simulink model "PLL_linecut"  (R2025a)
settings: Solver=FixedStepAuto  StartTime=0.0  StopTime=t_sim_start+t_end  FixedStep=Ts  RelTol=1e-3
values from neighbouring files (symbols this model uses):
  C_dc = 2.25    [PLLpara.m]
  Cf1 = 0.01    [PLLpara.m]
  Cf2 = 0.01    [PLLpara.m]
  dt_sag = t_c    [GFMPara.m]    (also in GFMPara_exp.m; PLLpara.m; VFMPara.m; VFMPara_exp.m)
  f_switching = 20e3    (= 20000)    [GFMPara_exp.m]    (also in PLLpara.m = 10000; VFMPara_exp.m)
  Id0 = Id    [PLLpara.m]
  Iq01 = 0    [PLLpara.m]
  Iq02 = (Ug*cos(asin((Xg*Id+Rg*Iq)/Ug))+Id*Rg-Iq*Xg)*Cf2+Iq    [PLLpara.m]
  ki_pll1 = ki    [PLLpara.m]
  kp_pll1 = kp    [PLLpara.m]
  Lc = 1e-9    (= 1e-09)    [GFMPara.m]    (also in GFMPara_exp.m; PLLpara.m; VFMPara.m; VFMPara_exp.m)
  Lf = 0.0592    [GFMPara.m]    (also in GFMPara_exp.m; PLLpara.m = 0.05; VFMPara.m = 0.05; VFMPara_exp.m = 0.05)
  Lg1 = X1    [PLLpara.m]    (also in VFMPara.m; VFMPara_exp.m)
  Lgg = Xgg    [PLLpara.m]    (also in VFMPara.m; VFMPara_exp.m)
  Rf = 1e-3    (= 0.001)    [PLLpara.m]
  Rg1 = R1    [PLLpara.m]    (also in VFMPara.m; VFMPara_exp.m = 4*R1/5)
  Rgg = Rgg    [PLLpara.m]    (also in VFMPara.m; VFMPara_exp.m)
  Sbase = 1    [GFMPara.m]    (also in GFMPara_exp.m; PLLpara.m; VFMPara.m; VFMPara_exp.m)
  t0 = t_sim_start +t_start    [PLLpara.m]    (also in VFMPara_exp.m)
  t0_sag = t_sim_start +t_start    [GFMPara.m]    (also in GFMPara_exp.m; PLLpara.m = 20; VFMPara.m; VFMPara_exp.m = 20)
  Tc = 1/f_switching    (= 5e-05)    [GFMPara_exp.m]    (also in PLLpara.m = 0.0001; VFMPara_exp.m)
  tc = t_c    [PLLpara.m]    (also in VFMPara_exp.m)
  Ts = 1/Fs    (= 1e-05)    [GFMPara.m]    (also in GFMPara_exp.m = 1e-06; PLLpara.m = 1e-06; VFMPara.m = 5e-06; VFMPara_exp.m = 1e-06)
  v_sag = Ug_fault    [GFMPara.m]    (also in GFMPara_exp.m; PLLpara.m; VFMPara.m; VFMPara_exp.m)
  Vbase = 1    [GFMPara.m]    (also in GFMPara_exp.m; PLLpara.m; VFMPara.m; VFMPara_exp.m)
  Vdc = 2.5    [PLLpara.m]
  w_i_GFL1 = 1100 *2*pi    (= 6911.5038379)    [PLLpara.m]
  w_i_GFL2 = 1100 *2*pi    (= 6911.5038379)    [PLLpara.m]
  w_pll1 = 10 *2*pi    (= 62.8318530718)    [PLLpara.m]
  w_tau1 = 1500 *2*pi    (= 9424.77796077)    [PLLpara.m]
  Wbase = 2*pi*50    (= 314.159265359)    [GFMPara.m]    (also in GFMPara_exp.m; PLLpara.m; VFMPara.m; VFMPara_exp.m)
  Zbase = Vbase/Ibase    (= 1)    [GFMPara.m]    (also in GFMPara_exp.m; PLLpara.m; VFMPara.m; VFMPara_exp.m)
undefined symbols (not defined in the file or in its folder): DiscIntNeverNeededParam, dspblkCoreblockFVToolHelper, gcbh, initial, position, postfault_SEP, sigbuilder_block, w_max, w_min, Ws
libraries: spsVoltageMeasurementLib x80, spsCurrentMeasurementLib x75, spsIdealSwitchLib x30, spsThreePhaseSeriesRLCBranchLib x21, spsControlledVoltageSourceLib x18, spsSeriesRLCBranchLib x14, powerlib_extras x10, spsHalfBridgeConverterLib x6, spsThreePhaseBreakerLib x6, spsDCVoltageSourceLib x4, simulink x3, spsThreePhaseFaultLib x3
(part 5 of 6)

== system PLL_linecut/Grid-Following Inverter (Simulink Block)3/inverter2 ==
  G : Inport
  block : Inport  Port=2
  Demux : Demux  Outputs=3
  NPC : Subsystem
  NPC1 : Subsystem
  NPC2 : Subsystem
  DC+ : PMIOPort  Tag=PMCPort  Side=Left
  N : PMIOPort  Tag=PMCPort  Port=2  Side=Left
  DC- : PMIOPort  Tag=PMCPort  Port=3  Side=Left
  A : PMIOPort  Tag=PMCPort  Port=4  Side=Right
  B : PMIOPort  Tag=PMCPort  Port=5  Side=Right
  C : PMIOPort  Tag=PMCPort  Port=6  Side=Right
  wires:
  G/1 -> Demux/1
  Demux/1 -> NPC/1(gate)
  Demux/2 -> NPC1/1(gate)
  Demux/3 -> NPC2/1(gate)
  block/1 -> NPC/2(block), NPC2/2(block), NPC1/2(block)
  connections:
  C/RConn1 -- NPC2/RConn1
  NPC1/RConn1 -- B/RConn1
  A/RConn1 -- NPC/RConn1
  DC+/RConn1 -- NPC2/LConn1 -- NPC1/LConn1 -- NPC/LConn1
  NPC/LConn3 -- NPC1/LConn3 -- NPC2/LConn3 -- DC-/RConn1
  NPC/LConn2 -- NPC2/LConn2 -- NPC1/LConn2 -- N/RConn1

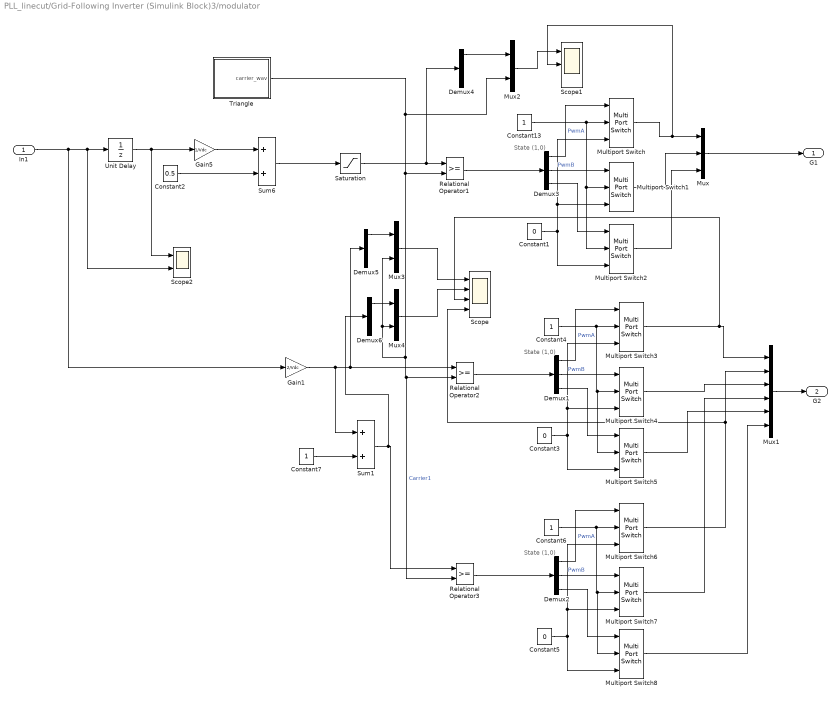
== system PLL_linecut/Grid-Following Inverter (Simulink Block)3/modulator ==
  note: State
      | (1,0)
  note: State
      | (1,0)
  note: State
      | (1,0)
  In1 : Inport  SampleTime=Ts
  Constant1 : Constant  Value=0
  Constant{4,6..7,13} (4 alike) : Constant
  Constant2 : Constant  Value=0.5
  Constant3 : Constant  Value=0
  Constant5 : Constant  Value=0
  Demux{1..6} (6 alike) : Demux  Outputs=3
      settings: DisplayOption=none
  Gain1 : Gain  Gain=2/Vdc
  Gain5 : Gain  Gain=1/Vdc
  Multiport Switch{,1..8} (9 alike) : MultiPortSwitch  DataPortOrder=Specify indices  DataPortIndices={1,0}  SaturateOnIntegerOverflow=off
  Mux : Mux  Inputs=[1 1 1]
  Mux1 : Mux  Inputs=6
  Mux2 : Mux  Inputs=2
  Mux3 : Mux  Inputs=2
  Mux4 : Mux  Inputs=2
  Relational Operator1 : RelationalOperator  OutDataTypeStr=float('double')
  Relational Operator2 : RelationalOperator  OutDataTypeStr=float('double')
  Relational Operator3 : RelationalOperator  OutDataTypeStr=float('double')
  Saturation : Saturate  UpperLimit=1  LowerLimit=0
  Scope : Scope  NumInputPorts=4
      settings: ActiveDisplayYMinimum=-0.88942  ActiveDisplayYMaximum=1.38183
  Scope1 : Scope  NumInputPorts=3
      settings: ActiveDisplayYMinimum=-0.044652738883298015  ActiveDisplayYMaximum=0.93484284042216537  DataLoggingVariableName=ScopeData6
  Scope2 : Scope  NumInputPorts=2
      settings: ActiveDisplayYMinimum=-0.80845  ActiveDisplayYMaximum=0.88075
  Sum1 : Sum  InputSameDT=on  SaturateOnIntegerOverflow=on  OutDataTypeStr=Inherit: Same as first input
  Sum6 : Sum  InputSameDT=on  SaturateOnIntegerOverflow=on  OutDataTypeStr=Inherit: Same as first input
  Triangle : Subsystem
  Unit Delay : UnitDelay  SampleTime=Tc  HasFrameUpgradeWarning=on
  G1 : Outport
  G2 : Outport  Port=2
  wires:
  Triangle/1(carrier_wav) -> Mux2/2, Mux4/2, Mux3/2, Relational Operator3/2, Relational Operator2/2, Relational Operator1/2  "Carrier1"
  Relational Operator1/1 -> Demux3/1
  Multiport Switch/1 -> Scope1/2, Mux/1
  Multiport Switch2/1 -> Mux/3
  Multiport Switch1/1 -> Mux/2
  Demux3/1 -> Multiport Switch/1  "PwmA"
  Demux3/2 -> Multiport Switch1/1  "PwmB"
  Demux3/3 -> Multiport Switch2/1
  Constant13/1 -> Multiport Switch2/2, Multiport Switch1/2, Multiport Switch/2
  Constant1/1 -> Multiport Switch1/3, Multiport Switch/3, Multiport Switch2/3
  Mux/1 -> G1/1
  Gain5/1 -> Sum6/1
  Constant2/1 -> Sum6/2
  In1/1 -> Scope2/2, Unit Delay/1, Gain1/1
  Demux1/3 -> Multiport Switch5/1
  Demux1/2 -> Multiport Switch4/1  "PwmB"
  Constant4/1 -> Multiport Switch5/2, Multiport Switch4/2, Multiport Switch3/2
  Multiport Switch5/1 -> Mux1/5
  Demux1/1 -> Multiport Switch3/1  "PwmA"
  Multiport Switch4/1 -> Mux1/3
  Constant3/1 -> Multiport Switch4/3, Multiport Switch3/3, Multiport Switch5/3
  Multiport Switch3/1 -> Scope/3, Mux1/1
  Relational Operator2/1 -> Demux1/1
  Constant5/1 -> Multiport Switch7/3, Multiport Switch6/3, Multiport Switch8/3
  Multiport Switch6/1 -> Scope/4, Mux1/2
  Constant6/1 -> Multiport Switch8/2, Multiport Switch7/2, Multiport Switch6/2
  Demux2/1 -> Multiport Switch6/1  "PwmA"
  Multiport Switch8/1 -> Mux1/6
  Multiport Switch7/1 -> Mux1/4
  Demux2/3 -> Multiport Switch8/1
  Demux2/2 -> Multiport Switch7/1  "PwmB"
  Relational Operator3/1 -> Demux2/1
  Gain1/1 -> Sum1/1, Demux5/1, Relational Operator2/1
  Constant7/1 -> Sum1/2
  Mux1/1 -> G2/1
  Sum1/1 -> Demux6/1, Relational Operator3/1
  Mux2/1 -> Scope1/1
  Demux4/1 -> Mux2/1
  Demux5/1 -> Mux3/1
  Demux6/1 -> Mux4/1
  Mux3/1 -> Scope/1
  Mux4/1 -> Scope/2
  Sum6/1 -> Saturation/1
  Saturation/1 -> Demux4/1, Relational Operator1/1
  Unit Delay/1 -> Scope2/1, Gain5/1

== system PLL_linecut/Grid-Following Inverter (Simulink Block)1/Current Controller/PI-DT-Estimated d ==
  enable : Inport
  reference : Inport  Port=2
  initial : Inport  Port=3
  actual : Inport  Port=4
  Discrete-Time Integrator : DiscreteIntegrator  gainval=1  ExternalReset=rising  InitialConditionSource=external  InitialCondition=initial  SampleTime=Ts  LimitOutput=on  UpperSaturationLimit=xmax  LowerSaturationLimit=xmin  ICPrevOutput=DiscIntNeverNeededParam  ICPrevScaledInput=DiscIntNeverNeededParam
  Ierror : Sum  Inputs=+-
  Ki : Gain  Gain=Ki  SaturateOnIntegerOverflow=on  OutDataTypeStr=Inherit: Same as input  ParamDataTypeStr=Inherit: Same as input
  Ki1 : Gain  Gain=Kg  SaturateOnIntegerOverflow=on  OutDataTypeStr=Inherit: Same as input  ParamDataTypeStr=Inherit: Same as input
  Kp : Gain  Gain=Kp  SaturateOnIntegerOverflow=on  OutDataTypeStr=Inherit: Same as input  ParamDataTypeStr=Inherit: Same as input
  Perror : Sum  Inputs=-+
  Product : Product  RndMeth=Zero
  Product1 : Product  RndMeth=Zero
  Product2 : Product  RndMeth=Zero
  Saturation : Saturate  UpperLimit=xmax  LowerLimit=xmin
  Scope4 : Scope  NumInputPorts=3
      settings: ActiveDisplayYMinimum=-3.25835  ActiveDisplayYMaximum=3.49302  DataLoggingVariableName=ScopeData10
  Sum1 : Sum  Inputs=+++  SaturateOnIntegerOverflow=on
  Out : Outport
  wires:
  Product1/1 -> Ki/1
  Ierror/1 -> Product1/1
  Product/1 -> Kp/1
  Perror/1 -> Product/1
  reference/1 -> Ierror/1, Perror/2
  actual/1 -> Ierror/2, Scope4/1, Perror/1
  initial/1 -> Product2/2, Discrete-Time Integrator/3
  enable/1 -> Product1/2, Product/2, Product2/1, Discrete-Time Integrator/2
  Discrete-Time Integrator/1 -> Scope4/2, Sum1/2
  Kp/1 -> Sum1/1
  Ki/1 -> Discrete-Time Integrator/1
  Sum1/1 -> Saturation/1
  Saturation/1 -> Scope4/3, Out/1
  Ki1/1 -> Sum1/3
  Product2/1 -> Ki1/1

== system PLL_linecut/Grid-Following Inverter (Simulink Block)1/Current Controller/PI-DT-Estimated q ==
  actual : Inport  SampleTime=Tc
  initial : Inport  Port=2  SampleTime=Tc
  reference : Inport  Port=3  SampleTime=Tc
  enable : Inport  Port=4  SampleTime=Tc
  Discrete-Time Integrator : DiscreteIntegrator  gainval=1  ExternalReset=rising  InitialConditionSource=external  InitialCondition=initial  SampleTime=Ts  LimitOutput=on  UpperSaturationLimit=xmax  LowerSaturationLimit=xmin  ICPrevOutput=DiscIntNeverNeededParam  ICPrevScaledInput=DiscIntNeverNeededParam
  Ierror : Sum  Inputs=+-
  Ki : Gain  Gain=Ki  SaturateOnIntegerOverflow=on  OutDataTypeStr=Inherit: Same as input  ParamDataTypeStr=Inherit: Same as input
  Ki1 : Gain  Gain=Kg  SaturateOnIntegerOverflow=on  OutDataTypeStr=Inherit: Same as input  ParamDataTypeStr=Inherit: Same as input
  Kp : Gain  Gain=Kp  SaturateOnIntegerOverflow=on  OutDataTypeStr=Inherit: Same as input  ParamDataTypeStr=Inherit: Same as input
  Perror : Sum  Inputs=-+
  Product : Product  RndMeth=Zero
  Product1 : Product  RndMeth=Zero
  Product2 : Product  RndMeth=Zero
  Saturation : Saturate  UpperLimit=xmax  LowerLimit=xmin
  Sum1 : Sum  Inputs=+++  SaturateOnIntegerOverflow=on
  Out : Outport
  wires:
  Product1/1 -> Ki/1
  Ierror/1 -> Product1/1
  Product/1 -> Kp/1
  Perror/1 -> Product/1
  reference/1 -> Ierror/1, Perror/2
  actual/1 -> Perror/1, Ierror/2
  initial/1 -> Product2/1, Discrete-Time Integrator/3
  enable/1 -> Product1/2, Product/2, Product2/2, Discrete-Time Integrator/2
  Discrete-Time Integrator/1 -> Sum1/2
  Kp/1 -> Sum1/1
  Ki/1 -> Discrete-Time Integrator/1
  Sum1/1 -> Saturation/1
  Saturation/1 -> Out/1
  Ki1/1 -> Sum1/3
  Product2/1 -> Ki1/1

== system PLL_linecut/Grid-Following Inverter (Simulink Block)1/LCL Filter/Anti-aliasing Filters (7)1 ==
  ABC : Inport  PortDimensions=3
  2nd-Order Filter : powerlib_extras/Discrete  Control Blocks/Discrete  2nd-Order Filter  FilterType=Lowpass  Fo=Fc  Zeta=0.707  Ts=Ts  Initialize=off  Vac_Init=[0.8 -25 60]  Vdc_Init=-0.4  PlotResponse=off  param1=[1 2000 0.2]
  2nd-Order Filter1 : powerlib_extras/Discrete  Control Blocks/Discrete  2nd-Order Filter  FilterType=Lowpass  Fo=Fc  Zeta=0.707  Ts=Ts  Initialize=off  Vac_Init=[0.8 -25 60]  Vdc_Init=-0.4  PlotResponse=off  param1=[1 5000 0.1]
  2nd-Order Filter2 : powerlib_extras/Discrete  Control Blocks/Discrete  2nd-Order Filter  FilterType=Lowpass  Fo=Fc  Zeta=0.707  Ts=Ts  Initialize=off  Vac_Init=[0.8 -25 60]  Vdc_Init=-0.4  PlotResponse=off  param1=[1 5000 0.1]
  Demux : Demux  Outputs=3
      settings: DisplayOption=none
  Mux : Mux  Inputs=3
  " ABC*" : Outport  VectorParamsAs1DForOutWhenUnconnected=off
  wires:
  Demux/2 -> 2nd-Order Filter1/1
  2nd-Order Filter1/1 -> Mux/2
  Mux/1 -> " ABC*"/1
  2nd-Order Filter/1 -> Mux/1
  ABC/1 -> Demux/1
  Demux/1 -> 2nd-Order Filter/1
  2nd-Order Filter2/1 -> Mux/3
  Demux/3 -> 2nd-Order Filter2/1

== system PLL_linecut/Grid-Following Inverter (Simulink Block)1/LCL Filter/Anti-aliasing Filters (7)3 ==
  ABC : Inport  PortDimensions=3
  Demux : Demux  Outputs=3
      settings: DisplayOption=none
  Mux : Mux  Inputs=3
  " ABC*" : Outport  VectorParamsAs1DForOutWhenUnconnected=off
  wires:
  Mux/1 -> " ABC*"/1
  ABC/1 -> Demux/1
  Demux/1 -> Mux/1
  Demux/2 -> Mux/2
  Demux/3 -> Mux/3

== system PLL_linecut/Grid-Following Inverter (Simulink Block)1/LCL Filter/LL -> LN1 ==
  note: Transformation from line-to-line voltage to line-to-neutral voltage.
      |
      | Author(s): Yitong Li
  In1 : Inport
  Fcn : Fcn  Expr=u[1]-u[3]
  Fcn1 : Fcn  Expr=u[2]-u[1]
  Fcn2 : Fcn  Expr=u[3]-u[2]
  Gain : Gain  Gain=1/3
  Mux9 : Mux  Inputs=3
  Out1 : Outport
  wires:
  In1/1 -> Gain/1
  Gain/1 -> Fcn/1, Fcn1/1, Fcn2/1
  Mux9/1 -> Out1/1
  Fcn2/1 -> Mux9/3
  Fcn1/1 -> Mux9/2
  Fcn/1 -> Mux9/1

== system PLL_linecut/Grid-Following Inverter (Simulink Block)1/LCL Filter/LL -> LN2 ==
  note: Transformation from line-to-line voltage to line-to-neutral voltage.
      |
      | Author(s): Yitong Li
  In1 : Inport
  Fcn : Fcn  Expr=u[1]-u[3]
  Fcn1 : Fcn  Expr=u[2]-u[1]
  Fcn2 : Fcn  Expr=u[3]-u[2]
  Gain : Gain  Gain=1/3
  Mux9 : Mux  Inputs=3
  Out1 : Outport
  wires:
  In1/1 -> Gain/1
  Gain/1 -> Fcn/1, Fcn1/1, Fcn2/1
  Mux9/1 -> Out1/1
  Fcn2/1 -> Mux9/3
  Fcn1/1 -> Mux9/2
  Fcn/1 -> Mux9/1

== system PLL_linecut/Grid-Following Inverter (Simulink Block)1/PLL (vabc -> vq)/Discrete PI ==
  note: Digital PI controller
      |
      | Author(s): Yitong Li
  enable : Inport  SampleTime=Tc
  reference : Inport  Port=2  SampleTime=Tc
  initial : Inport  Port=3  SampleTime=Tc
  actual : Inport  Port=4  SampleTime=Tc
  Discrete-Time Integrator : DiscreteIntegrator  gainval=1  ExternalReset=rising  InitialConditionSource=external  InitialCondition=initial  SampleTime=Tc  LimitOutput=on  UpperSaturationLimit=xmax  LowerSaturationLimit=xmin  ICPrevOutput=DiscIntNeverNeededParam  ICPrevScaledInput=DiscIntNeverNeededParam
  Ierror : Sum  Inputs=+-
  Ki : Gain  Gain=Ki  SaturateOnIntegerOverflow=on  OutDataTypeStr=Inherit: Same as input  ParamDataTypeStr=Inherit: Same as input
  Kp : Gain  Gain=Kp  SaturateOnIntegerOverflow=on  OutDataTypeStr=Inherit: Same as input  ParamDataTypeStr=Inherit: Same as input
  Perror : Sum  Inputs=-+
  Product : Product  RndMeth=Zero
  Product1 : Product  RndMeth=Zero
  Saturation : Saturate  UpperLimit=xmax  LowerLimit=xmin
  Scope : Scope  NumInputPorts=4
      settings: ActiveDisplayYMinimum=-0.3943  ActiveDisplayYMaximum=0.37329
  Sum : Sum  Inputs=|+-
  Sum1 : Sum  SaturateOnIntegerOverflow=on
  Sum2 : Sum  Inputs=|++
  Out : Outport  SampleTime=Tc
  tag scope: Xint2IBR_DSP=global
  wires:
  Product1/1 -> Ki/1
  Ierror/1 -> Product1/1
  Product/1 -> Kp/1
  Perror/1 -> Product/1
  actual/1 -> Perror/1, Ierror/2
  reference/1 -> Ierror/1, Perror/2
  enable/1 -> Sum/1, Product1/2, Product/2
  Discrete-Time Integrator/1 -> [Xint2IBR_DSP], Scope/2, Sum1/2
  Kp/1 -> Scope/1, Sum1/1
  Ki/1 -> Scope/3, Discrete-Time Integrator/1
  Sum1/1 -> Scope/4, Saturation/1
  Saturation/1 -> Out/1
  Sum/1 -> Discrete-Time Integrator/2
  Sum2/1 -> Discrete-Time Integrator/3
  initial/1 -> Sum2/1

== system PLL_linecut/Grid-Following Inverter (Simulink Block)1/PLL (vabc -> vq)/abc -> dq (Power-Invariant) ==
  note: Frame transformation from abc to dq.
      |
      | Author(s): Yitong Li
      |
      | Notes:
      |
      | The transformation is power-invariant.
      |
      | theta is the angle that d axis leads a axis.
      |
      | q axis leads d axis by 90 degrees.
  abc : Inport  SampleTime=Tc
  theta : Inport  Port=2  SampleTime=Tc
  ->d : Fcn  Expr=cos(u(4))*u(1) + cos(u(4)-2/3*pi)*u(2) + cos(u(4)-4/3*pi)*u(3)
  ->q : Fcn  Expr=-sin(u(4))*u(1) - sin(u(4)-2/3*pi)*u(2) - sin(u(4)-4/3*pi)*u(3)
  Gain : Gain  Gain=sqrt(2/3)
  Mux5 : Mux  Inputs=2
  Mux6 : Mux  Inputs=2
  dq : Outport  SampleTime=Tc
  wires:
  abc/1 -> Gain/1
  ->d/1 -> Mux6/1
  Gain/1 -> Mux5/1
  theta/1 -> Mux5/2
  ->q/1 -> Mux6/2
  Mux6/1 -> dq/1
  Mux5/1 -> ->d/1, ->q/1

== system PLL_linecut/Grid-Following Inverter (Simulink Block)1/inverter2/NPC ==
  gate : Inport
  block : Inport  Port=2
  Data Type Conversion{1..2,4..5} (4 alike) : DataTypeConversion  OutDataTypeStr=double  SaturateOnIntegerOverflow=off  RndMeth=Floor
  Data Type Conversion3 : DataTypeConversion  OutDataTypeStr=boolean  SaturateOnIntegerOverflow=off  RndMeth=Floor
  Data Type Conversion6 : DataTypeConversion  OutDataTypeStr=boolean  SaturateOnIntegerOverflow=off  RndMeth=Floor
  Demux : Demux  Outputs=2
  Ideal Switch{,1..3} (4 alike) : spsIdealSwitchLib/Ideal Switch  Ron=1e-6  Lon=0  IC=0  Rs=1e8  Cs=inf  Measurements=off
  Logical Operator : Logic  Operator=NOT  AllPortsSameDT=off  OutDataTypeStr=boolean
  Logical Operator1 : Logic  Operator=NOT  AllPortsSameDT=off  OutDataTypeStr=boolean
  Logical Operator{2,4..6} (4 alike) : Logic  AllPortsSameDT=off  OutDataTypeStr=float('double')
  Logical Operator3 : Logic  Operator=NOT  AllPortsSameDT=off  OutDataTypeStr=boolean
  Scope : Scope  NumInputPorts=3
      settings: ActiveDisplayYMinimum=-1  ActiveDisplayYMaximum=1  DataLoggingVariableName=ScopeData9
  Vbc1 : spsVoltageMeasurementLib/Voltage Measurement  PhasorSimulation=off  OutputType=Complex  PSBequivalent=0
  DC+ : PMIOPort  Tag=PMCPort  Side=Left
  N : PMIOPort  Tag=PMCPort  Port=2  Side=Left
  DC- : PMIOPort  Tag=PMCPort  Port=3  Side=Left
  out : PMIOPort  Tag=PMCPort  Port=4  Side=Right
  wires:
  Demux/1 -> Logical Operator2/1, Logical Operator/1
  Data Type Conversion6/1 -> Demux/1
  gate/1 -> Data Type Conversion6/1
  block/1 -> Data Type Conversion3/1
  Data Type Conversion3/1 -> Logical Operator3/1
  Logical Operator3/1 -> Logical Operator6/2, Logical Operator5/2, Logical Operator2/2, Logical Operator4/2
  Demux/2 -> Logical Operator5/1, Logical Operator1/1
  Data Type Conversion4/1 -> Scope/1, Ideal Switch/1
  Data Type Conversion1/1 -> Ideal Switch3/1
  Data Type Conversion5/1 -> Scope/2, Ideal Switch2/1
  Data Type Conversion2/1 -> Ideal Switch1/1
  Vbc1/1 -> Scope/3
  Logical Operator2/1 -> Data Type Conversion4/1
  Logical Operator/1 -> Logical Operator4/1
  Logical Operator4/1 -> Data Type Conversion1/1
  Logical Operator5/1 -> Data Type Conversion5/1
  Logical Operator6/1 -> Data Type Conversion2/1
  Logical Operator1/1 -> Logical Operator6/1
  connections:
  Ideal Switch1/RConn1 -- DC-/RConn1
  Ideal Switch/LConn1 -- DC+/RConn1
  Ideal Switch/RConn1 -- Ideal Switch3/RConn1 -- Vbc1/LConn1 -- out/RConn1 -- Ideal Switch1/LConn1
  Ideal Switch3/LConn1 -- Ideal Switch2/LConn1
  Ideal Switch2/RConn1 -- Vbc1/LConn2 -- N/RConn1

== system PLL_linecut/Grid-Following Inverter (Simulink Block)1/inverter2/NPC1 ==
  gate : Inport
  block : Inport  Port=2
  Data Type Conversion{1..2,4..5} (4 alike) : DataTypeConversion  OutDataTypeStr=double  SaturateOnIntegerOverflow=off  RndMeth=Floor
  Data Type Conversion3 : DataTypeConversion  OutDataTypeStr=boolean  SaturateOnIntegerOverflow=off  RndMeth=Floor
  Data Type Conversion6 : DataTypeConversion  OutDataTypeStr=boolean  SaturateOnIntegerOverflow=off  RndMeth=Floor
  Demux : Demux  Outputs=2
  Ideal Switch{,1..3} (4 alike) : spsIdealSwitchLib/Ideal Switch  Ron=1e-6  Lon=0  IC=0  Rs=1e8  Cs=inf  Measurements=off
  Logical Operator : Logic  Operator=NOT  AllPortsSameDT=off  OutDataTypeStr=boolean
  Logical Operator1 : Logic  Operator=NOT  AllPortsSameDT=off  OutDataTypeStr=boolean
  Logical Operator{2,4..6} (4 alike) : Logic  AllPortsSameDT=off  OutDataTypeStr=float('double')
  Logical Operator3 : Logic  Operator=NOT  AllPortsSameDT=off  OutDataTypeStr=boolean
  Scope : Scope  NumInputPorts=3
      settings: ActiveDisplayYMinimum=-1  ActiveDisplayYMaximum=1  DataLoggingVariableName=ScopeData9
  Vbc1 : spsVoltageMeasurementLib/Voltage Measurement  PhasorSimulation=off  OutputType=Complex  PSBequivalent=0
  DC+ : PMIOPort  Tag=PMCPort  Side=Left
  N : PMIOPort  Tag=PMCPort  Port=2  Side=Left
  DC- : PMIOPort  Tag=PMCPort  Port=3  Side=Left
  out : PMIOPort  Tag=PMCPort  Port=4  Side=Right
  wires:
  Demux/1 -> Logical Operator2/1, Logical Operator/1
  Data Type Conversion6/1 -> Demux/1
  gate/1 -> Data Type Conversion6/1
  block/1 -> Data Type Conversion3/1
  Data Type Conversion3/1 -> Logical Operator3/1
  Logical Operator3/1 -> Logical Operator6/2, Logical Operator5/2, Logical Operator2/2, Logical Operator4/2
  Demux/2 -> Logical Operator5/1, Logical Operator1/1
  Data Type Conversion4/1 -> Scope/1, Ideal Switch/1
  Data Type Conversion1/1 -> Ideal Switch3/1
  Data Type Conversion5/1 -> Scope/2, Ideal Switch2/1
  Data Type Conversion2/1 -> Ideal Switch1/1
  Vbc1/1 -> Scope/3
  Logical Operator2/1 -> Data Type Conversion4/1
  Logical Operator/1 -> Logical Operator4/1
  Logical Operator4/1 -> Data Type Conversion1/1
  Logical Operator5/1 -> Data Type Conversion5/1
  Logical Operator6/1 -> Data Type Conversion2/1
  Logical Operator1/1 -> Logical Operator6/1
  connections:
  Ideal Switch1/RConn1 -- DC-/RConn1
  Ideal Switch/LConn1 -- DC+/RConn1
  Ideal Switch1/LConn1 -- Ideal Switch3/RConn1 -- Ideal Switch/RConn1 -- out/RConn1 -- Vbc1/LConn1
  Ideal Switch3/LConn1 -- Ideal Switch2/LConn1
  N/RConn1 -- Ideal Switch2/RConn1 -- Vbc1/LConn2

== system PLL_linecut/Grid-Following Inverter (Simulink Block)1/inverter2/NPC2 ==
  gate : Inport
  block : Inport  Port=2
  Data Type Conversion{1..2,4..5} (4 alike) : DataTypeConversion  OutDataTypeStr=double  SaturateOnIntegerOverflow=off  RndMeth=Floor
  Data Type Conversion3 : DataTypeConversion  OutDataTypeStr=boolean  SaturateOnIntegerOverflow=off  RndMeth=Floor
  Data Type Conversion6 : DataTypeConversion  OutDataTypeStr=boolean  SaturateOnIntegerOverflow=off  RndMeth=Floor
  Demux : Demux  Outputs=2
  Ideal Switch{,1..3} (4 alike) : spsIdealSwitchLib/Ideal Switch  Ron=1e-6  Lon=0  IC=0  Rs=1e8  Cs=inf  Measurements=off
  Logical Operator : Logic  Operator=NOT  AllPortsSameDT=off  OutDataTypeStr=boolean
  Logical Operator1 : Logic  Operator=NOT  AllPortsSameDT=off  OutDataTypeStr=boolean
  Logical Operator{2,4..6} (4 alike) : Logic  AllPortsSameDT=off  OutDataTypeStr=float('double')
  Logical Operator3 : Logic  Operator=NOT  AllPortsSameDT=off  OutDataTypeStr=boolean
  Scope : Scope  NumInputPorts=3
      settings: ActiveDisplayYMinimum=-1  ActiveDisplayYMaximum=1  DataLoggingVariableName=ScopeData9
  Vbc1 : spsVoltageMeasurementLib/Voltage Measurement  PhasorSimulation=off  OutputType=Complex  PSBequivalent=0
  DC+ : PMIOPort  Tag=PMCPort  Side=Left
  N : PMIOPort  Tag=PMCPort  Port=2  Side=Left
  DC- : PMIOPort  Tag=PMCPort  Port=3  Side=Left
  out : PMIOPort  Tag=PMCPort  Port=4  Side=Right
  wires:
  Demux/1 -> Logical Operator2/1, Logical Operator/1
  Data Type Conversion6/1 -> Demux/1
  gate/1 -> Data Type Conversion6/1
  block/1 -> Data Type Conversion3/1
  Data Type Conversion3/1 -> Logical Operator3/1
  Logical Operator3/1 -> Logical Operator6/2, Logical Operator5/2, Logical Operator2/2, Logical Operator4/2
  Demux/2 -> Logical Operator5/1, Logical Operator1/1
  Data Type Conversion4/1 -> Scope/1, Ideal Switch/1
  Data Type Conversion1/1 -> Ideal Switch3/1
  Data Type Conversion5/1 -> Scope/2, Ideal Switch2/1
  Data Type Conversion2/1 -> Ideal Switch1/1
  Vbc1/1 -> Scope/3
  Logical Operator2/1 -> Data Type Conversion4/1
  Logical Operator/1 -> Logical Operator4/1
  Logical Operator4/1 -> Data Type Conversion1/1
  Logical Operator5/1 -> Data Type Conversion5/1
  Logical Operator6/1 -> Data Type Conversion2/1
  Logical Operator1/1 -> Logical Operator6/1
  connections:
  Ideal Switch1/RConn1 -- DC-/RConn1
  Ideal Switch/LConn1 -- DC+/RConn1
  Ideal Switch1/LConn1 -- Ideal Switch3/RConn1 -- Ideal Switch/RConn1 -- out/RConn1 -- Vbc1/LConn1
  Ideal Switch3/LConn1 -- Ideal Switch2/LConn1
  N/RConn1 -- Ideal Switch2/RConn1 -- Vbc1/LConn2

== system PLL_linecut/Grid-Following Inverter (Simulink Block)1/modulator/Triangle ==
  Constant1 : Constant  Value=0.5
  Constant2 : Constant  Value=-pi/2
  Constant4 : Constant  Value=2*pi
  Freq1 : Constant  Value=f_switching
  Freq2 : Constant  Value=2*pi
  Gain1 : Gain  Gain=1/pi  SaturateOnIntegerOverflow=on  OutDataTypeStr=Inherit: Same as input  ParamDataTypeStr=Inherit: Same as input
  Math Function : Math  Operator=mod  SignedPower=on
  Product : Product  Inputs=***  InputSameDT=on  SaturateOnIntegerOverflow=on  OutDataTypeStr=Inherit: Same as first input
  Sum : Sum  InputSameDT=on  SaturateOnIntegerOverflow=on  OutDataTypeStr=Inherit: Same as first input
  Sum1 : Sum  InputSameDT=on  SaturateOnIntegerOverflow=on  OutDataTypeStr=Inherit: Same as first input
  Trigonometric Function : Trigonometry  Operator=asin
  Trigonometric Function3 : Trigonometry
  t : DigitalClock  SampleTime=Ts
  carrier_wav : Outport
  wires:
  Trigonometric Function3/1 -> Trigonometric Function/1
  Trigonometric Function/1 -> Gain1/1
  Math Function/1 -> Trigonometric Function3/1
  Constant4/1 -> Math Function/2
  Freq1/1 -> Product/1
  Freq2/1 -> Product/3
  t/1 -> Product/2
  Gain1/1 -> Sum1/1
  Sum1/1 -> carrier_wav/1
  Constant1/1 -> Sum1/2
  Product/1 -> Sum/1
  Sum/1 -> Math Function/1
  Constant2/1 -> Sum/2

== system PLL_linecut/Grid-Following Inverter (Simulink Block)2/Current Controller/PI-DT-Estimated d ==
  enable : Inport
  reference : Inport  Port=2
  initial : Inport  Port=3
  actual : Inport  Port=4
  Discrete-Time Integrator : DiscreteIntegrator  gainval=1  ExternalReset=rising  InitialConditionSource=external  InitialCondition=initial  SampleTime=Ts  LimitOutput=on  UpperSaturationLimit=xmax  LowerSaturationLimit=xmin  ICPrevOutput=DiscIntNeverNeededParam  ICPrevScaledInput=DiscIntNeverNeededParam
  Ierror : Sum  Inputs=+-
  Ki : Gain  Gain=Ki  SaturateOnIntegerOverflow=on  OutDataTypeStr=Inherit: Same as input  ParamDataTypeStr=Inherit: Same as input
  Ki1 : Gain  Gain=Kg  SaturateOnIntegerOverflow=on  OutDataTypeStr=Inherit: Same as input  ParamDataTypeStr=Inherit: Same as input
  Kp : Gain  Gain=Kp  SaturateOnIntegerOverflow=on  OutDataTypeStr=Inherit: Same as input  ParamDataTypeStr=Inherit: Same as input
  Perror : Sum  Inputs=-+
  Product : Product  RndMeth=Zero
  Product1 : Product  RndMeth=Zero
  Product2 : Product  RndMeth=Zero
  Saturation : Saturate  UpperLimit=xmax  LowerLimit=xmin
  Sum1 : Sum  Inputs=+++  SaturateOnIntegerOverflow=on
  Out : Outport
  wires:
  Product1/1 -> Ki/1
  Ierror/1 -> Product1/1
  Product/1 -> Kp/1
  Perror/1 -> Product/1
  reference/1 -> Ierror/1, Perror/2
  actual/1 -> Ierror/2, Perror/1
  initial/1 -> Product2/2, Discrete-Time Integrator/3
  enable/1 -> Product1/2, Product/2, Product2/1, Discrete-Time Integrator/2
  Discrete-Time Integrator/1 -> Sum1/2
  Kp/1 -> Sum1/1
  Ki/1 -> Discrete-Time Integrator/1
  Sum1/1 -> Saturation/1
  Saturation/1 -> Out/1
  Ki1/1 -> Sum1/3
  Product2/1 -> Ki1/1

== system PLL_linecut/Grid-Following Inverter (Simulink Block)2/Current Controller/PI-DT-Estimated q ==
  actual : Inport
  initial : Inport  Port=2
  reference : Inport  Port=3
  enable : Inport  Port=4
  Discrete-Time Integrator : DiscreteIntegrator  gainval=1  ExternalReset=rising  InitialConditionSource=external  InitialCondition=initial  SampleTime=Ts  LimitOutput=on  UpperSaturationLimit=xmax  LowerSaturationLimit=xmin  ICPrevOutput=DiscIntNeverNeededParam  ICPrevScaledInput=DiscIntNeverNeededParam
  Ierror : Sum  Inputs=+-
  Ki : Gain  Gain=Ki  SaturateOnIntegerOverflow=on  OutDataTypeStr=Inherit: Same as input  ParamDataTypeStr=Inherit: Same as input
  Ki1 : Gain  Gain=Kg  SaturateOnIntegerOverflow=on  OutDataTypeStr=Inherit: Same as input  ParamDataTypeStr=Inherit: Same as input
  Kp : Gain  Gain=Kp  SaturateOnIntegerOverflow=on  OutDataTypeStr=Inherit: Same as input  ParamDataTypeStr=Inherit: Same as input
  Perror : Sum  Inputs=-+
  Product : Product  RndMeth=Zero
  Product1 : Product  RndMeth=Zero
  Product2 : Product  RndMeth=Zero
  Saturation : Saturate  UpperLimit=xmax  LowerLimit=xmin
  Sum1 : Sum  Inputs=+++  SaturateOnIntegerOverflow=on
  Out : Outport
  wires:
  Product1/1 -> Ki/1
  Ierror/1 -> Product1/1
  Product/1 -> Kp/1
  Perror/1 -> Product/1
  reference/1 -> Ierror/1, Perror/2
  actual/1 -> Perror/1, Ierror/2
  initial/1 -> Product2/2, Discrete-Time Integrator/3
  enable/1 -> Product1/2, Product/2, Product2/1, Discrete-Time Integrator/2
  Discrete-Time Integrator/1 -> Sum1/2
  Kp/1 -> Sum1/1
  Ki/1 -> Discrete-Time Integrator/1
  Sum1/1 -> Saturation/1
  Saturation/1 -> Out/1
  Ki1/1 -> Sum1/3
  Product2/1 -> Ki1/1

== system PLL_linecut/Grid-Following Inverter (Simulink Block)2/LCL Filter/LL -> LN1 ==
  note: Transformation from line-to-line voltage to line-to-neutral voltage.
      |
      | Author(s): Yitong Li
  In1 : Inport
  Fcn : Fcn  Expr=u[1]-u[3]
  Fcn1 : Fcn  Expr=u[2]-u[1]
  Fcn2 : Fcn  Expr=u[3]-u[2]
  Gain : Gain  Gain=1/3
  Mux9 : Mux  Inputs=3
  Out1 : Outport
  wires:
  In1/1 -> Gain/1
  Gain/1 -> Fcn/1, Fcn1/1, Fcn2/1
  Mux9/1 -> Out1/1
  Fcn2/1 -> Mux9/3
  Fcn1/1 -> Mux9/2
  Fcn/1 -> Mux9/1

== system PLL_linecut/Grid-Following Inverter (Simulink Block)2/LCL Filter/LL -> LN2 ==
  note: Transformation from line-to-line voltage to line-to-neutral voltage.
      |
      | Author(s): Yitong Li
  In1 : Inport
  Fcn : Fcn  Expr=u[1]-u[3]
  Fcn1 : Fcn  Expr=u[2]-u[1]
  Fcn2 : Fcn  Expr=u[3]-u[2]
  Gain : Gain  Gain=1/3
  Mux9 : Mux  Inputs=3
  Out1 : Outport
  wires:
  In1/1 -> Gain/1
  Gain/1 -> Fcn/1, Fcn1/1, Fcn2/1
  Mux9/1 -> Out1/1
  Fcn2/1 -> Mux9/3
  Fcn1/1 -> Mux9/2
  Fcn/1 -> Mux9/1

== system PLL_linecut/Grid-Following Inverter (Simulink Block)2/PLL (vabc -> vq)/Discrete PI ==
  note: Digital PI controller
      |
      | Author(s): Yitong Li
  enable : Inport
  reference : Inport  Port=2
  initial : Inport  Port=3
  actual : Inport  Port=4
  Discrete-Time Integrator : DiscreteIntegrator  gainval=1  ExternalReset=rising  InitialConditionSource=external  InitialCondition=initial  SampleTime=Ts  LimitOutput=on  UpperSaturationLimit=xmax  LowerSaturationLimit=xmin  ICPrevOutput=DiscIntNeverNeededParam  ICPrevScaledInput=DiscIntNeverNeededParam
  Ierror : Sum  Inputs=+-
  Ki : Gain  Gain=Ki  SaturateOnIntegerOverflow=on  OutDataTypeStr=Inherit: Same as input  ParamDataTypeStr=Inherit: Same as input
  Kp : Gain  Gain=Kp  SaturateOnIntegerOverflow=on  OutDataTypeStr=Inherit: Same as input  ParamDataTypeStr=Inherit: Same as input
  Perror : Sum  Inputs=-+
  Product : Product  RndMeth=Zero
  Product1 : Product  RndMeth=Zero
  Saturation : Saturate  UpperLimit=xmax  LowerLimit=xmin
  Scope : Scope  NumInputPorts=4
      settings: ActiveDisplayYMinimum=-47.13559  ActiveDisplayYMaximum=50.05528
  Step : Step  Time=3  After=-66.86  SampleTime=0
  Sum : Sum  Inputs=|+-
  Sum1 : Sum  SaturateOnIntegerOverflow=on
  Sum2 : Sum  Inputs=|++
  Voltage Sag1 : Subsystem  AncestorBlock=SimplusGT/Single Pulse  mask{t0=30, dt=dt_sag, Am=v_sag}
      mask prompts: t0 "t0 (s), starting time"; dt "dt (s), pulse width"; Am "Am, pulse amplitude"
  Out : Outport
  tag scope: Xint1IBR=global
  wires:
  Product1/1 -> Ki/1
  Ierror/1 -> Product1/1
  Product/1 -> Kp/1
  Perror/1 -> Product/1
  actual/1 -> Perror/1, Ierror/2
  reference/1 -> Ierror/1, Perror/2
  enable/1 -> Sum/1, Product1/2, Product/2
  Discrete-Time Integrator/1 -> Scope/2, Sum1/2, [Xint1IBR]
  Kp/1 -> Scope/1, Sum1/1
  Ki/1 -> Discrete-Time Integrator/1
  Sum1/1 -> Saturation/1
  Saturation/1 -> Out/1
  Sum/1 -> Scope/3, Discrete-Time Integrator/2
  Sum2/1 -> Discrete-Time Integrator/3
  initial/1 -> Sum2/1
  Step/1 -> Sum2/2
  Voltage Sag1/1(Out) -> Sum/2

== system PLL_linecut/Grid-Following Inverter (Simulink Block)2/PLL (vabc -> vq)/abc -> dq (Power-Invariant) ==
  note: Frame transformation from abc to dq.
      |
      | Author(s): Yitong Li
      |
      | Notes:
      |
      | The transformation is power-invariant.
      |
      | theta is the angle that d axis leads a axis.
      |
      | q axis leads d axis by 90 degrees.
  abc : Inport
  theta : Inport  Port=2
  ->d : Fcn  Expr=cos(u(4))*u(1) + cos(u(4)-2/3*pi)*u(2) + cos(u(4)-4/3*pi)*u(3)
  ->q : Fcn  Expr=-sin(u(4))*u(1) - sin(u(4)-2/3*pi)*u(2) - sin(u(4)-4/3*pi)*u(3)
  Gain : Gain  Gain=sqrt(2/3)
  Mux5 : Mux  Inputs=2
  Mux6 : Mux  Inputs=2
  dq : Outport
  wires:
  abc/1 -> Gain/1
  ->d/1 -> Mux6/1
  Gain/1 -> Mux5/1
  theta/1 -> Mux5/2
  ->q/1 -> Mux6/2
  Mux6/1 -> dq/1
  Mux5/1 -> ->d/1, ->q/1

== system PLL_linecut/Grid-Following Inverter (Simulink Block)3/Current Controller/PI-DT-Estimated d ==
  enable : Inport
  reference : Inport  Port=2
  initial : Inport  Port=3
  actual : Inport  Port=4
  Discrete-Time Integrator : DiscreteIntegrator  gainval=1  ExternalReset=rising  InitialConditionSource=external  InitialCondition=initial  SampleTime=Ts  LimitOutput=on  UpperSaturationLimit=xmax  LowerSaturationLimit=xmin  ICPrevOutput=DiscIntNeverNeededParam  ICPrevScaledInput=DiscIntNeverNeededParam
  Ierror : Sum  Inputs=+-
  Ki : Gain  Gain=Ki  SaturateOnIntegerOverflow=on  OutDataTypeStr=Inherit: Same as input  ParamDataTypeStr=Inherit: Same as input
  Ki1 : Gain  Gain=Kg  SaturateOnIntegerOverflow=on  OutDataTypeStr=Inherit: Same as input  ParamDataTypeStr=Inherit: Same as input
  Kp : Gain  Gain=Kp  SaturateOnIntegerOverflow=on  OutDataTypeStr=Inherit: Same as input  ParamDataTypeStr=Inherit: Same as input
  Perror : Sum  Inputs=-+
  Product : Product  RndMeth=Zero
  Product1 : Product  RndMeth=Zero
  Product2 : Product  RndMeth=Zero
  Saturation : Saturate  UpperLimit=xmax  LowerLimit=xmin
  Scope4 : Scope  NumInputPorts=3
      settings: ActiveDisplayYMinimum=-3.25835  ActiveDisplayYMaximum=3.49302  DataLoggingVariableName=ScopeData10
  Sum1 : Sum  Inputs=+++  SaturateOnIntegerOverflow=on
  Out : Outport
  wires:
  Product1/1 -> Ki/1
  Ierror/1 -> Product1/1
  Product/1 -> Kp/1
  Perror/1 -> Product/1
  reference/1 -> Ierror/1, Perror/2
  actual/1 -> Ierror/2, Scope4/1, Perror/1
  initial/1 -> Product2/2, Discrete-Time Integrator/3
  enable/1 -> Product1/2, Product/2, Product2/1, Discrete-Time Integrator/2
  Discrete-Time Integrator/1 -> Scope4/2, Sum1/2
  Kp/1 -> Sum1/1
  Ki/1 -> Discrete-Time Integrator/1
  Sum1/1 -> Saturation/1
  Saturation/1 -> Scope4/3, Out/1
  Ki1/1 -> Sum1/3
  Product2/1 -> Ki1/1

== system PLL_linecut/Grid-Following Inverter (Simulink Block)3/Current Controller/PI-DT-Estimated q ==
  actual : Inport  SampleTime=Tc
  initial : Inport  Port=2  SampleTime=Tc
  reference : Inport  Port=3  SampleTime=Tc
  enable : Inport  Port=4  SampleTime=Tc
  Discrete-Time Integrator : DiscreteIntegrator  gainval=1  ExternalReset=rising  InitialConditionSource=external  InitialCondition=initial  SampleTime=Ts  LimitOutput=on  UpperSaturationLimit=xmax  LowerSaturationLimit=xmin  ICPrevOutput=DiscIntNeverNeededParam  ICPrevScaledInput=DiscIntNeverNeededParam
  Ierror : Sum  Inputs=+-
  Ki : Gain  Gain=Ki  SaturateOnIntegerOverflow=on  OutDataTypeStr=Inherit: Same as input  ParamDataTypeStr=Inherit: Same as input
  Ki1 : Gain  Gain=Kg  SaturateOnIntegerOverflow=on  OutDataTypeStr=Inherit: Same as input  ParamDataTypeStr=Inherit: Same as input
  Kp : Gain  Gain=Kp  SaturateOnIntegerOverflow=on  OutDataTypeStr=Inherit: Same as input  ParamDataTypeStr=Inherit: Same as input
  Perror : Sum  Inputs=-+
  Product : Product  RndMeth=Zero
  Product1 : Product  RndMeth=Zero
  Product2 : Product  RndMeth=Zero
  Saturation : Saturate  UpperLimit=xmax  LowerLimit=xmin
  Sum1 : Sum  Inputs=+++  SaturateOnIntegerOverflow=on
  Out : Outport
  wires:
  Product1/1 -> Ki/1
  Ierror/1 -> Product1/1
  Product/1 -> Kp/1
  Perror/1 -> Product/1
  reference/1 -> Ierror/1, Perror/2
  actual/1 -> Perror/1, Ierror/2
  initial/1 -> Product2/1, Discrete-Time Integrator/3
  enable/1 -> Product1/2, Product/2, Product2/2, Discrete-Time Integrator/2
  Discrete-Time Integrator/1 -> Sum1/2
  Kp/1 -> Sum1/1
  Ki/1 -> Discrete-Time Integrator/1
  Sum1/1 -> Saturation/1
  Saturation/1 -> Out/1
  Ki1/1 -> Sum1/3
  Product2/1 -> Ki1/1

== system PLL_linecut/Grid-Following Inverter (Simulink Block)3/LCL Filter/Anti-aliasing Filters (7)1 ==
  ABC : Inport  PortDimensions=3
  2nd-Order Filter : powerlib_extras/Discrete  Control Blocks/Discrete  2nd-Order Filter  FilterType=Lowpass  Fo=Fc  Zeta=0.707  Ts=Ts  Initialize=off  Vac_Init=[0.8 -25 60]  Vdc_Init=-0.4  PlotResponse=off  param1=[1 2000 0.2]
  2nd-Order Filter1 : powerlib_extras/Discrete  Control Blocks/Discrete  2nd-Order Filter  FilterType=Lowpass  Fo=Fc  Zeta=0.707  Ts=Ts  Initialize=off  Vac_Init=[0.8 -25 60]  Vdc_Init=-0.4  PlotResponse=off  param1=[1 5000 0.1]
  2nd-Order Filter2 : powerlib_extras/Discrete  Control Blocks/Discrete  2nd-Order Filter  FilterType=Lowpass  Fo=Fc  Zeta=0.707  Ts=Ts  Initialize=off  Vac_Init=[0.8 -25 60]  Vdc_Init=-0.4  PlotResponse=off  param1=[1 5000 0.1]
  Demux : Demux  Outputs=3
      settings: DisplayOption=none
  Mux : Mux  Inputs=3
  " ABC*" : Outport  VectorParamsAs1DForOutWhenUnconnected=off
  wires:
  Demux/2 -> 2nd-Order Filter1/1
  2nd-Order Filter1/1 -> Mux/2
  Mux/1 -> " ABC*"/1
  2nd-Order Filter/1 -> Mux/1
  ABC/1 -> Demux/1
  Demux/1 -> 2nd-Order Filter/1
  2nd-Order Filter2/1 -> Mux/3
  Demux/3 -> 2nd-Order Filter2/1

== system PLL_linecut/Grid-Following Inverter (Simulink Block)3/LCL Filter/Anti-aliasing Filters (7)3 ==
  ABC : Inport  PortDimensions=3
  Demux : Demux  Outputs=3
      settings: DisplayOption=none
  Mux : Mux  Inputs=3
  " ABC*" : Outport  VectorParamsAs1DForOutWhenUnconnected=off
  wires:
  Mux/1 -> " ABC*"/1
  ABC/1 -> Demux/1
  Demux/1 -> Mux/1
  Demux/2 -> Mux/2
  Demux/3 -> Mux/3

== system PLL_linecut/Grid-Following Inverter (Simulink Block)3/LCL Filter/LL -> LN1 ==
  note: Transformation from line-to-line voltage to line-to-neutral voltage.
      |
      | Author(s): Yitong Li
  In1 : Inport
  Fcn : Fcn  Expr=u[1]-u[3]
  Fcn1 : Fcn  Expr=u[2]-u[1]
  Fcn2 : Fcn  Expr=u[3]-u[2]
  Gain : Gain  Gain=1/3
  Mux9 : Mux  Inputs=3
  Out1 : Outport
  wires:
  In1/1 -> Gain/1
  Gain/1 -> Fcn/1, Fcn1/1, Fcn2/1
  Mux9/1 -> Out1/1
  Fcn2/1 -> Mux9/3
  Fcn1/1 -> Mux9/2
  Fcn/1 -> Mux9/1

== system PLL_linecut/Grid-Following Inverter (Simulink Block)3/LCL Filter/LL -> LN2 ==
  note: Transformation from line-to-line voltage to line-to-neutral voltage.
      |
      | Author(s): Yitong Li
  In1 : Inport
  Fcn : Fcn  Expr=u[1]-u[3]
  Fcn1 : Fcn  Expr=u[2]-u[1]
  Fcn2 : Fcn  Expr=u[3]-u[2]
  Gain : Gain  Gain=1/3
  Mux9 : Mux  Inputs=3
  Out1 : Outport
  wires:
  In1/1 -> Gain/1
  Gain/1 -> Fcn/1, Fcn1/1, Fcn2/1
  Mux9/1 -> Out1/1
  Fcn2/1 -> Mux9/3
  Fcn1/1 -> Mux9/2
  Fcn/1 -> Mux9/1

== system PLL_linecut/Grid-Following Inverter (Simulink Block)3/PLL (vabc -> vq)/Discrete PI ==
  note: Digital PI controller
      |
      | Author(s): Yitong Li
  enable : Inport  SampleTime=Tc
  reference : Inport  Port=2  SampleTime=Tc
  initial : Inport  Port=3  SampleTime=Tc
  actual : Inport  Port=4  SampleTime=Tc
  Discrete-Time Integrator : DiscreteIntegrator  gainval=1  ExternalReset=rising  InitialConditionSource=external  InitialCondition=initial  SampleTime=Tc  LimitOutput=on  UpperSaturationLimit=xmax  LowerSaturationLimit=xmin  ICPrevOutput=DiscIntNeverNeededParam  ICPrevScaledInput=DiscIntNeverNeededParam
  Ierror : Sum  Inputs=+-
  Ki : Gain  Gain=Ki  SaturateOnIntegerOverflow=on  OutDataTypeStr=Inherit: Same as input  ParamDataTypeStr=Inherit: Same as input
  Kp : Gain  Gain=Kp  SaturateOnIntegerOverflow=on  OutDataTypeStr=Inherit: Same as input  ParamDataTypeStr=Inherit: Same as input
  Perror : Sum  Inputs=-+
  Product : Product  RndMeth=Zero
  Product1 : Product  RndMeth=Zero
  Saturation : Saturate  UpperLimit=xmax  LowerLimit=xmin
  Scope : Scope  NumInputPorts=4
      settings: ActiveDisplayYMinimum=-0.3943  ActiveDisplayYMaximum=0.37329
  Sum : Sum  Inputs=|+-
  Sum1 : Sum  SaturateOnIntegerOverflow=on
  Sum2 : Sum  Inputs=|++
  Out : Outport  SampleTime=Tc
  tag scope: Xint2IBR_DSP=global
  wires:
  Product1/1 -> Ki/1
  Ierror/1 -> Product1/1
  Product/1 -> Kp/1
  Perror/1 -> Product/1
  actual/1 -> Perror/1, Ierror/2
  reference/1 -> Ierror/1, Perror/2
  enable/1 -> Sum/1, Product1/2, Product/2
  Discrete-Time Integrator/1 -> [Xint2IBR_DSP], Scope/2, Sum1/2
  Kp/1 -> Scope/1, Sum1/1
  Ki/1 -> Scope/3, Discrete-Time Integrator/1
  Sum1/1 -> Scope/4, Saturation/1
  Saturation/1 -> Out/1
  Sum/1 -> Discrete-Time Integrator/2
  Sum2/1 -> Discrete-Time Integrator/3
  initial/1 -> Sum2/1

== system PLL_linecut/Grid-Following Inverter (Simulink Block)3/PLL (vabc -> vq)/abc -> dq (Power-Invariant) ==
  note: Frame transformation from abc to dq.
      |
      | Author(s): Yitong Li
      |
      | Notes:
      |
      | The transformation is power-invariant.
      |
      | theta is the angle that d axis leads a axis.
      |
      | q axis leads d axis by 90 degrees.
  abc : Inport  SampleTime=Tc
  theta : Inport  Port=2  SampleTime=Tc
  ->d : Fcn  Expr=cos(u(4))*u(1) + cos(u(4)-2/3*pi)*u(2) + cos(u(4)-4/3*pi)*u(3)
  ->q : Fcn  Expr=-sin(u(4))*u(1) - sin(u(4)-2/3*pi)*u(2) - sin(u(4)-4/3*pi)*u(3)
  Gain : Gain  Gain=sqrt(2/3)
  Mux5 : Mux  Inputs=2
  Mux6 : Mux  Inputs=2
  dq : Outport  SampleTime=Tc
  wires:
  abc/1 -> Gain/1
  ->d/1 -> Mux6/1
  Gain/1 -> Mux5/1
  theta/1 -> Mux5/2
  ->q/1 -> Mux6/2
  Mux6/1 -> dq/1
  Mux5/1 -> ->d/1, ->q/1

== system PLL_linecut/Grid-Following Inverter (Simulink Block)3/inverter2/NPC ==
  gate : Inport
  block : Inport  Port=2
  Data Type Conversion{1..2,4..5} (4 alike) : DataTypeConversion  OutDataTypeStr=double  SaturateOnIntegerOverflow=off  RndMeth=Floor
  Data Type Conversion3 : DataTypeConversion  OutDataTypeStr=boolean  SaturateOnIntegerOverflow=off  RndMeth=Floor
  Data Type Conversion6 : DataTypeConversion  OutDataTypeStr=boolean  SaturateOnIntegerOverflow=off  RndMeth=Floor
  Demux : Demux  Outputs=2
  Ideal Switch{,1..3} (4 alike) : spsIdealSwitchLib/Ideal Switch  Ron=1e-6  Lon=0  IC=0  Rs=1e8  Cs=inf  Measurements=off
  Logical Operator : Logic  Operator=NOT  AllPortsSameDT=off  OutDataTypeStr=boolean
  Logical Operator1 : Logic  Operator=NOT  AllPortsSameDT=off  OutDataTypeStr=boolean
  Logical Operator{2,4..6} (4 alike) : Logic  AllPortsSameDT=off  OutDataTypeStr=float('double')
  Logical Operator3 : Logic  Operator=NOT  AllPortsSameDT=off  OutDataTypeStr=boolean
  Scope : Scope  NumInputPorts=3
      settings: ActiveDisplayYMinimum=-1  ActiveDisplayYMaximum=1  DataLoggingVariableName=ScopeData9
  Vbc1 : spsVoltageMeasurementLib/Voltage Measurement  PhasorSimulation=off  OutputType=Complex  PSBequivalent=0
  DC+ : PMIOPort  Tag=PMCPort  Side=Left
  N : PMIOPort  Tag=PMCPort  Port=2  Side=Left
  DC- : PMIOPort  Tag=PMCPort  Port=3  Side=Left
  out : PMIOPort  Tag=PMCPort  Port=4  Side=Right
  wires:
  Demux/1 -> Logical Operator2/1, Logical Operator/1
  Data Type Conversion6/1 -> Demux/1
  gate/1 -> Data Type Conversion6/1
  block/1 -> Data Type Conversion3/1
  Data Type Conversion3/1 -> Logical Operator3/1
  Logical Operator3/1 -> Logical Operator6/2, Logical Operator5/2, Logical Operator2/2, Logical Operator4/2
  Demux/2 -> Logical Operator5/1, Logical Operator1/1
  Data Type Conversion4/1 -> Scope/1, Ideal Switch/1
  Data Type Conversion1/1 -> Ideal Switch3/1
  Data Type Conversion5/1 -> Scope/2, Ideal Switch2/1
  Data Type Conversion2/1 -> Ideal Switch1/1
  Vbc1/1 -> Scope/3
  Logical Operator2/1 -> Data Type Conversion4/1
  Logical Operator/1 -> Logical Operator4/1
  Logical Operator4/1 -> Data Type Conversion1/1
  Logical Operator5/1 -> Data Type Conversion5/1
  Logical Operator6/1 -> Data Type Conversion2/1
  Logical Operator1/1 -> Logical Operator6/1
  connections:
  Ideal Switch1/RConn1 -- DC-/RConn1
  Ideal Switch/LConn1 -- DC+/RConn1
  Ideal Switch/RConn1 -- Ideal Switch3/RConn1 -- Vbc1/LConn1 -- out/RConn1 -- Ideal Switch1/LConn1
  Ideal Switch3/LConn1 -- Ideal Switch2/LConn1
  Ideal Switch2/RConn1 -- Vbc1/LConn2 -- N/RConn1

== system PLL_linecut/Grid-Following Inverter (Simulink Block)3/inverter2/NPC1 ==
  gate : Inport
  block : Inport  Port=2
  Data Type Conversion{1..2,4..5} (4 alike) : DataTypeConversion  OutDataTypeStr=double  SaturateOnIntegerOverflow=off  RndMeth=Floor
  Data Type Conversion3 : DataTypeConversion  OutDataTypeStr=boolean  SaturateOnIntegerOverflow=off  RndMeth=Floor
  Data Type Conversion6 : DataTypeConversion  OutDataTypeStr=boolean  SaturateOnIntegerOverflow=off  RndMeth=Floor
  Demux : Demux  Outputs=2
  Ideal Switch{,1..3} (4 alike) : spsIdealSwitchLib/Ideal Switch  Ron=1e-6  Lon=0  IC=0  Rs=1e8  Cs=inf  Measurements=off
  Logical Operator : Logic  Operator=NOT  AllPortsSameDT=off  OutDataTypeStr=boolean
  Logical Operator1 : Logic  Operator=NOT  AllPortsSameDT=off  OutDataTypeStr=boolean
  Logical Operator{2,4..6} (4 alike) : Logic  AllPortsSameDT=off  OutDataTypeStr=float('double')
  Logical Operator3 : Logic  Operator=NOT  AllPortsSameDT=off  OutDataTypeStr=boolean
  Scope : Scope  NumInputPorts=3
      settings: ActiveDisplayYMinimum=-1  ActiveDisplayYMaximum=1  DataLoggingVariableName=ScopeData9
  Vbc1 : spsVoltageMeasurementLib/Voltage Measurement  PhasorSimulation=off  OutputType=Complex  PSBequivalent=0
  DC+ : PMIOPort  Tag=PMCPort  Side=Left
  N : PMIOPort  Tag=PMCPort  Port=2  Side=Left
  DC- : PMIOPort  Tag=PMCPort  Port=3  Side=Left
  out : PMIOPort  Tag=PMCPort  Port=4  Side=Right
  wires:
  Demux/1 -> Logical Operator2/1, Logical Operator/1
  Data Type Conversion6/1 -> Demux/1
  gate/1 -> Data Type Conversion6/1
  block/1 -> Data Type Conversion3/1
  Data Type Conversion3/1 -> Logical Operator3/1
  Logical Operator3/1 -> Logical Operator6/2, Logical Operator5/2, Logical Operator2/2, Logical Operator4/2
  Demux/2 -> Logical Operator5/1, Logical Operator1/1
  Data Type Conversion4/1 -> Scope/1, Ideal Switch/1
  Data Type Conversion1/1 -> Ideal Switch3/1
  Data Type Conversion5/1 -> Scope/2, Ideal Switch2/1
  Data Type Conversion2/1 -> Ideal Switch1/1
  Vbc1/1 -> Scope/3
  Logical Operator2/1 -> Data Type Conversion4/1
  Logical Operator/1 -> Logical Operator4/1
  Logical Operator4/1 -> Data Type Conversion1/1
  Logical Operator5/1 -> Data Type Conversion5/1
  Logical Operator6/1 -> Data Type Conversion2/1
  Logical Operator1/1 -> Logical Operator6/1
  connections:
  Ideal Switch1/RConn1 -- DC-/RConn1
  Ideal Switch/LConn1 -- DC+/RConn1
  Ideal Switch1/LConn1 -- Ideal Switch3/RConn1 -- Ideal Switch/RConn1 -- out/RConn1 -- Vbc1/LConn1
  Ideal Switch3/LConn1 -- Ideal Switch2/LConn1
  N/RConn1 -- Ideal Switch2/RConn1 -- Vbc1/LConn2

== system PLL_linecut/Grid-Following Inverter (Simulink Block)3/inverter2/NPC2 ==
  gate : Inport
  block : Inport  Port=2
  Data Type Conversion{1..2,4..5} (4 alike) : DataTypeConversion  OutDataTypeStr=double  SaturateOnIntegerOverflow=off  RndMeth=Floor
  Data Type Conversion3 : DataTypeConversion  OutDataTypeStr=boolean  SaturateOnIntegerOverflow=off  RndMeth=Floor
  Data Type Conversion6 : DataTypeConversion  OutDataTypeStr=boolean  SaturateOnIntegerOverflow=off  RndMeth=Floor
  Demux : Demux  Outputs=2
  Ideal Switch{,1..3} (4 alike) : spsIdealSwitchLib/Ideal Switch  Ron=1e-6  Lon=0  IC=0  Rs=1e8  Cs=inf  Measurements=off
  Logical Operator : Logic  Operator=NOT  AllPortsSameDT=off  OutDataTypeStr=boolean
  Logical Operator1 : Logic  Operator=NOT  AllPortsSameDT=off  OutDataTypeStr=boolean
  Logical Operator{2,4..6} (4 alike) : Logic  AllPortsSameDT=off  OutDataTypeStr=float('double')
  Logical Operator3 : Logic  Operator=NOT  AllPortsSameDT=off  OutDataTypeStr=boolean
  Scope : Scope  NumInputPorts=3
      settings: ActiveDisplayYMinimum=-1  ActiveDisplayYMaximum=1  DataLoggingVariableName=ScopeData9
  Vbc1 : spsVoltageMeasurementLib/Voltage Measurement  PhasorSimulation=off  OutputType=Complex  PSBequivalent=0
  DC+ : PMIOPort  Tag=PMCPort  Side=Left
  N : PMIOPort  Tag=PMCPort  Port=2  Side=Left
  DC- : PMIOPort  Tag=PMCPort  Port=3  Side=Left
  out : PMIOPort  Tag=PMCPort  Port=4  Side=Right
  wires:
  Demux/1 -> Logical Operator2/1, Logical Operator/1
  Data Type Conversion6/1 -> Demux/1
  gate/1 -> Data Type Conversion6/1
  block/1 -> Data Type Conversion3/1
  Data Type Conversion3/1 -> Logical Operator3/1
  Logical Operator3/1 -> Logical Operator6/2, Logical Operator5/2, Logical Operator2/2, Logical Operator4/2
  Demux/2 -> Logical Operator5/1, Logical Operator1/1
  Data Type Conversion4/1 -> Scope/1, Ideal Switch/1
  Data Type Conversion1/1 -> Ideal Switch3/1
  Data Type Conversion5/1 -> Scope/2, Ideal Switch2/1
  Data Type Conversion2/1 -> Ideal Switch1/1
  Vbc1/1 -> Scope/3
  Logical Operator2/1 -> Data Type Conversion4/1
  Logical Operator/1 -> Logical Operator4/1
  Logical Operator4/1 -> Data Type Conversion1/1
  Logical Operator5/1 -> Data Type Conversion5/1
  Logical Operator6/1 -> Data Type Conversion2/1
  Logical Operator1/1 -> Logical Operator6/1
  connections:
  Ideal Switch1/RConn1 -- DC-/RConn1
  Ideal Switch/LConn1 -- DC+/RConn1
  Ideal Switch1/LConn1 -- Ideal Switch3/RConn1 -- Ideal Switch/RConn1 -- out/RConn1 -- Vbc1/LConn1
  Ideal Switch3/LConn1 -- Ideal Switch2/LConn1
  N/RConn1 -- Ideal Switch2/RConn1 -- Vbc1/LConn2
